simulink model "EHB_MOTOR"  (R2023b)
settings: Solver=FixedStepDiscrete  StartTime=0.0  StopTime=inf  FixedStep=0.0001  RelTol=1e-3  EnableMultiTasking=on
undefined symbols (not defined in the file): CAN_EHB_VCU0x125, CAN_EHB_VCU0x126, CAN_id0x120_Data, Cos_Table, Cos_Table1, EHB_DTC_status, R, Sin_BreakPoint, Sin_BreakPoint1, Sin_Table, Sin_Table1, T
libraries: simulink x30
(part 8 of 9)

== stateflow chart EHB_MOTOR/EHB_MOTOR_PRO/DIAG/MotLockDiag/ErrorSignalCount ==
  state errClear
    en:Mot_locked_err=0;
    Counter=0;
  state errConfirm
    en:Mot_locked_err=0;
    du:Counter++;
  state errTrue
    en:Mot_locked_err=1;
    Counter=0;
  (default) -> errClear
  errClear -> errConfirm : [Mot_locked==1]
  errConfirm -> errClear [order 2] : [Mot_locked==0]
  errTrue -> errClear : [Recover==1]
  errConfirm -> errTrue [order 1] : [Counter >= tiMotLocked_C]
  data: Mot_locked input boolean; Mot_locked_err output boolean; tiMotLocked_C input uint16; Counter local uint16; Recover input uint8

== stateflow chart EHB_MOTOR/EHB_MOTOR_PRO/MODE/Chart1 ==
  (default) -> (junction 5)
  (junction 5) -> (junction 7) [order 1] : [input]
  (junction 5) -> (junction 23) [order 2] : {ZeroCal_cnt=0;}
  (junction 7) -> (junction 9) : {ZeroCal_cnt++;}
  (junction 9) -> (junction 13) [order 1] : [ZeroCal_cnt>=9000]
  (junction 9) -> (junction 20) [order 2]
  (junction 13) -> (junction 15) : {Zero_Angle=MOT_Angle;
      | ZeroCal_cmplt=1;}
  (junction 20) -> (junction 23)
  (junction 15) -> (junction 20)
  data: MOT_Angle input uint16; input input boolean; ZeroCal_cnt local uint16; Zero_Angle output uint16; ZeroCal_cmplt output boolean

== stateflow chart EHB_MOTOR/EHB_MOTOR_PRO/DIAG/UDS_interface/DTC_pack ==
  (default) -> (junction 15) : %12v欠压故障
  (junction 15) -> (junction 17) [order 1] : [minBAT == 1]
  (junction 15) -> (junction 25) [order 2] : {EHB_DTC[12]&=0x01;}
  (junction 17) -> (junction 20) : {EHB_DTC[12]|=0x03;}
  (junction 25) -> (junction 20)
  (junction 20) -> (junction 30) [order 1] : [Clear_minBAT_req == 1]
  (junction 20) -> (junction 34) [order 2]
  (junction 30) -> (junction 32) : {EHB_DTC[12]&=0x02;}
  (junction 34) -> (junction 32)
  (junction 32) -> (junction 66) : %12v过压故障
  (junction 66) -> (junction 68) [order 1] : [maxBAT == 1]
  (junction 66) -> (junction 72) [order 2] : {EHB_DTC[13]&=0x01;}
  (junction 68) -> (junction 70) : {EHB_DTC[13]|=0x03;}
  (junction 72) -> (junction 70)
  (junction 70) -> (junction 78) [order 1] : [Clear_minBAT_req == 1]
  (junction 70) -> (junction 80) [order 2]
  (junction 78) -> (junction 75) : {EHB_DTC[13]&=0x02;}
  (junction 80) -> (junction 75)
  (junction 75) -> (junction 97) : %过温故障
  (junction 97) -> (junction 91) [order 1] : [overTemp == 1]
  (junction 97) -> (junction 95) [order 2] : {EHB_DTC[10]&=0x01;}
  (junction 91) -> (junction 89) : {EHB_DTC[10]|=0x03;}
  (junction 95) -> (junction 89)
  (junction 89) -> (junction 87) [order 1] : [Clear_minBAT_req == 1]
  (junction 89) -> (junction 83) [order 2]
  (junction 87) -> (junction 94) : {EHB_DTC[10]&=0x02;}
  (junction 83) -> (junction 94)
  (junction 94) -> (junction 103) : %温度传感器故障
  (junction 103) -> (junction 108) [order 1] : [errTempSensor == 1]
  (junction 103) -> (junction 106) [order 2] : {EHB_DTC[15]&=0x01;}
  (junction 108) -> (junction 105) : {EHB_DTC[15]|=0x03;}
  (junction 106) -> (junction 105)
  (junction 105) -> (junction 112) [order 1] : [Clear_minBAT_req == 1]
  (junction 105) -> (junction 115) [order 2]
  (junction 112) -> (junction 104) : {EHB_DTC[15]&=0x02;}
  (junction 115) -> (junction 104)
  (junction 104) -> (junction 127) : %过流故障
  (junction 127) -> (junction 131) [order 1] : [overCurrent == 1]
  (junction 127) -> (junction 124) [order 2] : {EHB_DTC[11]&=0x01;}
  (junction 131) -> (junction 118) : {EHB_DTC[11]|=0x03;}
  (junction 124) -> (junction 118)
  (junction 118) -> (junction 123) [order 1] : [Clear_minBAT_req == 1]
  (junction 118) -> (junction 129) [order 2]
  (junction 123) -> (junction 128) : {EHB_DTC[11]&=0x02;}
  (junction 129) -> (junction 128)
  (junction 128) -> (junction 140) : %电流传感器故障
  (junction 140) -> (junction 145) [order 1] : [errCurSensor == 1]
  (junction 140) -> (junction 148) [order 2] : {EHB_DTC[14]&=0x01;}
  (junction 145) -> (junction 138) : {EHB_DTC[14]|=0x03;}
  (junction 148) -> (junction 138)
  (junction 138) -> (junction 135) [order 1] : [Clear_minBAT_req == 1]
  (junction 138) -> (junction 141) [order 2]
  (junction 135) -> (junction 147) : {EHB_DTC[14]&=0x02;}
  (junction 141) -> (junction 147)
  (junction 147) -> (junction 162) : %角度传感器信号错误故障
  (junction 162) -> (junction 151) [order 1] : [errAngleSensor == 1]
  (junction 162) -> (junction 153) [order 2] : {EHB_DTC[0]&=0x01;}
  (junction 151) -> (junction 157) : {EHB_DTC[0]|=0x03;}
  (junction 153) -> (junction 157)
  (junction 157) -> (junction 164) [order 1] : [Clear_minBAT_req == 1]
  (junction 157) -> (junction 154) [order 2]
  (junction 164) -> (junction 150) : {EHB_DTC[0]&=0x02;}
  (junction 154) -> (junction 150)
  (junction 150) -> (junction 168) : %角度传感器没有信号故障
  (junction 168) -> (junction 175) [order 1] : [noAngleSensor == 1]
  (junction 168) -> (junction 173) [order 2] : {EHB_DTC[1]&=0x01;}
  (junction 175) -> (junction 169) : {EHB_DTC[1]|=0x03;}
  (junction 173) -> (junction 169)
  (junction 169) -> (junction 174) [order 1] : [Clear_minBAT_req == 1]
  (junction 169) -> (junction 176) [order 2]
  (junction 174) -> (junction 180) : {EHB_DTC[1]&=0x02;}
  (junction 176) -> (junction 180)
  (junction 180) -> (junction 183) : %角度传感器没有标定故障
  (junction 183) -> (junction 193) [order 1] : [unCalAngleSensor == 1]
  (junction 183) -> (junction 195) [order 2] : {EHB_DTC[2]&=0x01;}
  (junction 193) -> (junction 185) : {EHB_DTC[2]|=0x03;}
  (junction 195) -> (junction 185)
  (junction 185) -> (junction 188) [order 1] : [Clear_minBAT_req == 1]
  (junction 185) -> (junction 190) [order 2]
  (junction 188) -> (junction 191) : {EHB_DTC[2]&=0x02;}
  (junction 190) -> (junction 191)
  (junction 191) -> (junction 208) : %压力传感器信号错误故障
  (junction 208) -> (junction 205) [order 1] : [errPreSensor == 1]
  (junction 208) -> (junction 198) [order 2] : {EHB_DTC[3]&=0x01;}
  (junction 205) -> (junction 209) : {EHB_DTC[3]|=0x03;}
  (junction 198) -> (junction 209)
  (junction 209) -> (junction 200) [order 1] : [Clear_minBAT_req == 1]
  (junction 209) -> (junction 207) [order 2]
  (junction 200) -> (junction 199) : {EHB_DTC[3]&=0x02;}
  (junction 207) -> (junction 199)
  (junction 199) -> (junction 218) : %压力传感器没有信号故障
  (junction 218) -> (junction 216) [order 1] : [noPreSensor == 1]
  (junction 218) -> (junction 228) [order 2] : {EHB_DTC[4]&=0x01;}
  (junction 216) -> (junction 215) : {EHB_DTC[4]|=0x03;}
  (junction 228) -> (junction 215)
  (junction 215) -> (junction 224) [order 1] : [Clear_minBAT_req == 1]
  (junction 215) -> (junction 221) [order 2]
  (junction 224) -> (junction 220) : {EHB_DTC[4]&=0x02;}
  (junction 221) -> (junction 220)
  (junction 220) -> (junction 238) : %压力传感器没有标定故障
  (junction 238) -> (junction 235) [order 1] : [unCalPreSensor == 1]
  (junction 238) -> (junction 230) [order 2] : {EHB_DTC[5]&=0x01;}
  (junction 235) -> (junction 239) : {EHB_DTC[5]|=0x03;}
  (junction 230) -> (junction 239)
  (junction 239) -> (junction 233) [order 1] : [Clear_minBAT_req == 1]
  (junction 239) -> (junction 234) [order 2]
  (junction 233) -> (junction 242) : {EHB_DTC[5]&=0x02;}
  (junction 234) -> (junction 242)
  (junction 242) -> (junction 248) : %扭矩传感器信号错误故障
  (junction 248) -> (junction 256) [order 1] : [errTqSensor == 1]
  (junction 248) -> (junction 259) [order 2] : {EHB_DTC[6]&=0x01;}
  (junction 256) -> (junction 251) : {EHB_DTC[6]|=0x03;}
  (junction 259) -> (junction 251)
  (junction 251) -> (junction 257) [order 1] : [Clear_minBAT_req == 1]
  (junction 251) -> (junction 252) [order 2]
  (junction 257) -> (junction 246) : {EHB_DTC[6]&=0x02;}
  (junction 252) -> (junction 246)
  (junction 246) -> (junction 276) : %扭矩传感器没有信号故障
  (junction 276) -> (junction 273) [order 1] : [noTqSensor == 1]
  (junction 276) -> (junction 268) [order 2] : {EHB_DTC[7]&=0x01;}
  (junction 273) -> (junction 269) : {EHB_DTC[7]|=0x03;}
  (junction 268) -> (junction 269)
  (junction 269) -> (junction 264) [order 1] : [Clear_minBAT_req == 1]
  (junction 269) -> (junction 270) [order 2]
  (junction 264) -> (junction 274) : {EHB_DTC[7]&=0x02;}
  (junction 270) -> (junction 274)
  (junction 274) -> (junction 289) : %扭矩传感器没有标定故障
  (junction 289) -> (junction 279) [order 1] : [unCalTqSensor == 1]
  (junction 289) -> (junction 288) [order 2] : {EHB_DTC[8]&=0x01;}
  (junction 279) -> (junction 285) : {EHB_DTC[8]|=0x03;}
  (junction 288) -> (junction 285)
  (junction 285) -> (junction 290) [order 1] : [Clear_minBAT_req == 1]
  (junction 285) -> (junction 283) [order 2]
  (junction 290) -> (junction 280) : {EHB_DTC[8]&=0x02;}
  (junction 283) -> (junction 280)
  (junction 280) -> (junction 295) : %电机回路故障
  (junction 295) -> (junction 304) [order 1] : [errMotorloop == 1]
  (junction 295) -> (junction 305) [order 2] : {EHB_DTC[9]&=0x01;}
  (junction 304) -> (junction 298) : {EHB_DTC[9]|=0x03;}
  (junction 305) -> (junction 298)
  (junction 298) -> (junction 297) [order 1] : [Clear_minBAT_req == 1]
  (junction 298) -> (junction 299) [order 2]
  (junction 297) -> (junction 306) : {EHB_DTC[9]&=0x02;}
  (junction 299) -> (junction 306)
  (junction 306) -> (junction 323) : %预充电路故障
  (junction 323) -> (junction 316) [order 1] : [errPreCtl == 1]
  (junction 323) -> (junction 315) [order 2] : {EHB_DTC[16]&=0x01;}
  (junction 316) -> (junction 318) : {EHB_DTC[16]|=0x03;}
  (junction 315) -> (junction 318)
  (junction 318) -> (junction 321) [order 1] : [Clear_minBAT_req == 1]
  (junction 318) -> (junction 314) [order 2]
  (junction 321) -> (junction 319) : {EHB_DTC[16]&=0x02;}
  (junction 314) -> (junction 319)
  (junction 319) -> (junction 326) : %5v输出电路故障
  (junction 326) -> (junction 337) [order 1] : [err5vOUT == 1]
  (junction 326) -> (junction 335) [order 2] : {EHB_DTC[17]&=0x01;}
  (junction 337) -> (junction 333) : {EHB_DTC[17]|=0x03;}
  (junction 335) -> (junction 333)
  (junction 333) -> (junction 329) [order 1] : [Clear_minBAT_req == 1]
  (junction 333) -> (junction 334) [order 2]
  (junction 329) -> (junction 328) : {EHB_DTC[17]&=0x02;}
  (junction 334) -> (junction 328)
  (junction 328) -> (junction 356) : %高边输出电路1故障
  (junction 356) -> (junction 348) [order 1] : [errHSO1 == 1]
  (junction 356) -> (junction 352) [order 2] : {EHB_DTC[18]&=0x01;}
  (junction 348) -> (junction 349) : {EHB_DTC[18]|=0x03;}
  (junction 352) -> (junction 349)
  (junction 349) -> (junction 346) [order 1] : [Clear_minBAT_req == 1]
  (junction 349) -> (junction 345) [order 2]
  (junction 346) -> (junction 350) : {EHB_DTC[18]&=0x02;}
  (junction 345) -> (junction 350)
  (junction 350) -> (junction 358) : %高边输出电路2故障
  (junction 358) -> (junction 363) [order 1] : [errHSO2 == 1]
  (junction 358) -> (junction 368) [order 2] : {EHB_DTC[19]&=0x01;}
  (junction 363) -> (junction 371) : {EHB_DTC[19]|=0x03;}
  (junction 368) -> (junction 371)
  (junction 371) -> (junction 372) [order 1] : [Clear_minBAT_req == 1]
  (junction 371) -> (junction 366) [order 2]
  (junction 372) -> (junction 362) : {EHB_DTC[19]&=0x02;}
  (junction 366) -> (junction 362)
  (junction 362) -> (junction 386) : %A3941芯片故障
  (junction 386) -> (junction 382) [order 1] : [errA3941 == 1]
  (junction 386) -> (junction 376) [order 2] : {EHB_DTC[20]&=0x01;}
  (junction 382) -> (junction 377) : {EHB_DTC[20]|=0x03;}
  (junction 376) -> (junction 377)
  (junction 377) -> (junction 388) [order 1] : [Clear_minBAT_req == 1]
  (junction 377) -> (junction 379) [order 2]
  (junction 388) -> (junction 385) : {EHB_DTC[20]&=0x02;}
  (junction 379) -> (junction 385)
  (junction 385) -> (junction 392) : %占空比发送电路故障
  (junction 392) -> (junction 403) [order 1] : [errPWM == 1]
  (junction 392) -> (junction 404) [order 2] : {EHB_DTC[21]&=0x01;}
  (junction 403) -> (junction 394) : {EHB_DTC[21]|=0x03;}
  (junction 404) -> (junction 394)
  (junction 394) -> (junction 390) [order 1] : [Clear_minBAT_req == 1]
  (junction 394) -> (junction 393) [order 2]
  (junction 390) -> (junction 397) : {EHB_DTC[21]&=0x02;}
  (junction 393) -> (junction 397)
  (junction 397) -> (junction 419) : %电机响应状态异常故障
  (junction 419) -> (junction 406) [order 1] : [errResponce == 1]
  (junction 419) -> (junction 418) [order 2] : {EHB_DTC[22]&=0x01;}
  (junction 406) -> (junction 409) : {EHB_DTC[22]|=0x03;}
  (junction 418) -> (junction 409)
  (junction 409) -> (junction 420) [order 1] : [Clear_minBAT_req == 1]
  (junction 409) -> (junction 408) [order 2]
  (junction 420) -> (junction 410) : {EHB_DTC[22]&=0x02;}
  (junction 408) -> (junction 410)
  (junction 410) -> (junction 422) : %CAN收发器电路故障
  (junction 422) -> (junction 434) [order 1] : [errCANHW == 1]
  (junction 422) -> (junction 423) [order 2] : {EHB_DTC[23]&=0x01;}
  (junction 434) -> (junction 430) : {EHB_DTC[23]|=0x03;}
  (junction 423) -> (junction 430)
  (junction 430) -> (junction 436) [order 1] : [Clear_minBAT_req == 1]
  (junction 430) -> (junction 429) [order 2]
  (junction 436) -> (junction 425) : {EHB_DTC[23]&=0x02;}
  (junction 429) -> (junction 425)
  (junction 425) -> (junction 442) : %CAN数据丢失故障
  (junction 442) -> (junction 446) [order 1] : [CANDataLoss == 1]
  (junction 442) -> (junction 440) [order 2] : {EHB_DTC[24]&=0x01;}
  (junction 446) -> (junction 451) : {EHB_DTC[24]|=0x03;}
  (junction 440) -> (junction 451)
  (junction 451) -> (junction 450) [order 1] : [Clear_minBAT_req == 1]
  (junction 451) -> (junction 445) [order 2]
  (junction 450) -> (junction 438) : {EHB_DTC[24]&=0x02;}
  (junction 445) -> (junction 438)
  (junction 438) -> (junction 462) : %CAN BUSOFF
  (junction 462) -> (junction 466) [order 1] : [BUSOFF == 1]
  (junction 462) -> (junction 468) [order 2] : {EHB_DTC[25]&=0x01;}
  (junction 466) -> (junction 455) : {EHB_DTC[25]|=0x03;}
  (junction 468) -> (junction 455)
  (junction 455) -> (junction 456) [order 1] : [Clear_minBAT_req == 1]
  (junction 455) -> (junction 459) [order 2]
  (junction 456) -> (junction 463) : {EHB_DTC[25]&=0x02;}
  (junction 459) -> (junction 463)
  (junction 463) -> (junction 476) : %Tracker2对地短路故障
  (junction 476) -> (junction 506) [order 1] : [Tracker2_Short2GND_err == 1]
  (junction 476) -> (junction 520) [order 2] : {EHB_DTC[26]&=0x01;}
  (junction 506) -> (junction 474) : {EHB_DTC[26]|=0x03;}
  (junction 520) -> (junction 474)
  (junction 474) -> (junction 511) [order 1] : [Clear_minBAT_req == 1]
  (junction 474) -> (junction 499) [order 2]
  (junction 511) -> (junction 473) : {EHB_DTC[26]&=0x02;}
  (junction 499) -> (junction 473)
  (junction 473) -> (junction 522) : %Tracker2过压故障
  (junction 522) -> (junction 518) [order 1] : [Tracker2_OverVolt_err == 1]
  (junction 522) -> (junction 519) [order 2] : {EHB_DTC[27]&=0x01;}
  (junction 518) -> (junction 500) : {EHB_DTC[27]|=0x03;}
  (junction 519) -> (junction 500)
  (junction 500) -> (junction 501) [order 1] : [Clear_minBAT_req == 1]
  (junction 500) -> (junction 510) [order 2]
  (junction 501) -> (junction 471) : {EHB_DTC[27]&=0x02;}
  (junction 510) -> (junction 471)
  (junction 471) -> (junction 515) : %Tracker2欠压故障
  (junction 515) -> (junction 512) [order 1] : [Tracker2_UnderVolt_err == 1]
  (junction 515) -> (junction 502) [order 2] : {EHB_DTC[28]&=0x01;}
  (junction 512) -> (junction 503) : {EHB_DTC[28]|=0x03;}
  (junction 502) -> (junction 503)
  (junction 503) -> (junction 472) [order 1] : [Clear_minBAT_req == 1]
  (junction 503) -> (junction 514) [order 2]
  (junction 472) -> (junction 484) : {EHB_DTC[28]&=0x02;}
  (junction 514) -> (junction 484)
  (junction 484) -> (junction 509) : %Tracker1对地短路故障
  (junction 509) -> (junction 513) [order 1] : [Tracker1_Short2GND_err == 1]
  (junction 509) -> (junction 521) [order 2] : {EHB_DTC[29]&=0x01;}
  (junction 513) -> (junction 508) : {EHB_DTC[29]|=0x03;}
  (junction 521) -> (junction 508)
  (junction 508) -> (junction 523) [order 1] : [Clear_minBAT_req == 1]
  (junction 508) -> (junction 491) [order 2]
  (junction 523) -> (junction 516) : {EHB_DTC[29]&=0x02;}
  (junction 491) -> (junction 516)
  (junction 516) -> (junction 517) : %Tracker1过压故障
  (junction 517) -> (junction 504) [order 1] : [Tracker1_OverVolt_err == 1]
  (junction 517) -> (junction 524) [order 2] : {EHB_DTC[30]&=0x01;}
  (junction 504) -> (junction 470) : {EHB_DTC[30]|=0x03;}
  (junction 524) -> (junction 470)
  (junction 470) -> (junction 494) [order 1] : [Clear_minBAT_req == 1]
  (junction 470) -> (junction 505) [order 2]
  (junction 494) -> (junction 496) : {EHB_DTC[30]&=0x02;}
  (junction 505) -> (junction 496)
  (junction 496) -> (junction 485) : %Tracker1欠压故障
  (junction 485) -> (junction 507) [order 1] : [Tracker1_UnderVolt_err == 1]
  (junction 485) -> (junction 475) [order 2] : {EHB_DTC[31]&=0x01;}
  (junction 507) -> (junction 492) : {EHB_DTC[31]|=0x03;}
  (junction 475) -> (junction 492)
  (junction 492) -> (junction 477) [order 1] : [Clear_minBAT_req == 1]
  (junction 492) -> (junction 478) [order 2]
  (junction 477) -> (junction 479) : {EHB_DTC[31]&=0x02;}
  (junction 478) -> (junction 479)
  (junction 479) -> (junction 480) : %Voltage reference对地短路故障
  (junction 480) -> (junction 481) [order 1] : [VltRef_Short2GND_err == 1]
  (junction 480) -> (junction 497) [order 2] : {EHB_DTC[32]&=0x01;}
  (junction 481) -> (junction 482) : {EHB_DTC[32]|=0x03;}
  (junction 497) -> (junction 482)
  (junction 482) -> (junction 486) [order 1] : [Clear_minBAT_req == 1]
  (junction 482) -> (junction 483) [order 2]
  (junction 486) -> (junction 487) : {EHB_DTC[32]&=0x02;}
  (junction 483) -> (junction 487)
  (junction 487) -> (junction 493) : %Voltage reference过压故障
  (junction 493) -> (junction 488) [order 1] : [VltRef_OverVolt_err == 1]
  (junction 493) -> (junction 489) [order 2] : {EHB_DTC[33]&=0x01;}
  (junction 488) -> (junction 490) : {EHB_DTC[33]|=0x03;}
  (junction 489) -> (junction 490)
  (junction 490) -> (junction 495) [order 1] : [Clear_minBAT_req == 1]
  (junction 490) -> (junction 498) [order 2]
  (junction 495) -> (junction 553) : {EHB_DTC[33]&=0x02;}
  (junction 498) -> (junction 553)
  (junction 553) -> (junction 537) : %Voltage reference欠压故障
  (junction 537) -> (junction 554) [order 1] : [VltRef_UnderVolt_err == 1]
  (junction 537) -> (junction 587) [order 2] : {EHB_DTC[34]&=0x01;}
  (junction 554) -> (junction 582) : {EHB_DTC[34]|=0x03;}
  (junction 587) -> (junction 582)
  (junction 582) -> (junction 576) [order 1] : [Clear_minBAT_req == 1]
  (junction 582) -> (junction 539) [order 2]
  (junction 576) -> (junction 568) : {EHB_DTC[34]&=0x02;}
  (junction 539) -> (junction 568)
  (junction 568) -> (junction 556) : %Communication LDO对地短路故障
  (junction 556) -> (junction 583) [order 1] : [CommuLDO_Short2GND_err == 1]
  (junction 556) -> (junction 541) [order 2] : {EHB_DTC[35]&=0x01;}
  (junction 583) -> (junction 562) : {EHB_DTC[35]|=0x03;}
  (junction 541) -> (junction 562)
  (junction 562) -> (junction 555) [order 1] : [Clear_minBAT_req == 1]
  (junction 562) -> (junction 560) [order 2]
  (junction 555) -> (junction 532) : {EHB_DTC[35]&=0x02;}
  (junction 560) -> (junction 532)
  (junction 532) -> (junction 579) : %Communication LDO过压故障
  (junction 579) -> (junction 540) [order 1] : [CommuLDO_OverVolt_err == 1]
  (junction 579) -> (junction 558) [order 2] : {EHB_DTC[36]&=0x01;}
  (junction 540) -> (junction 570) : {EHB_DTC[36]|=0x03;}
  (junction 558) -> (junction 570)
  (junction 570) -> (junction 584) [order 1] : [Clear_minBAT_req == 1]
  (junction 570) -> (junction 561) [order 2]
  (junction 584) -> (junction 557) : {EHB_DTC[36]&=0x02;}
  (junction 561) -> (junction 557)
  (junction 557) -> (junction 552) : %Communication LDO欠压故障
  (junction 552) -> (junction 547) [order 1] : [CommuLDO_UnderVolt_err == 1]
  (junction 552) -> (junction 563) [order 2] : {EHB_DTC[37]&=0x01;}
  (junction 547) -> (junction 559) : {EHB_DTC[37]|=0x03;}
  (junction 563) -> (junction 559)
  (junction 559) -> (junction 564) [order 1] : [Clear_minBAT_req == 1]
  (junction 559) -> (junction 573) [order 2]
  (junction 564) -> (junction 586) : {EHB_DTC[37]&=0x02;}
  (junction 573) -> (junction 586)
  (junction 586) -> (junction 535) : %Core voltage对地短路故障
  (junction 535) -> (junction 581) [order 1] : [CoreVlt_Short2GND_err == 1]
  (junction 535) -> (junction 585) [order 2] : {EHB_DTC[38]&=0x01;}
  (junction 581) -> (junction 549) : {EHB_DTC[38]|=0x03;}
  (junction 585) -> (junction 549)
  (junction 549) -> (junction 565) [order 1] : [Clear_minBAT_req == 1]
  (junction 549) -> (junction 551) [order 2]
  (junction 565) -> (junction 542) : {EHB_DTC[38]&=0x02;}
  (junction 551) -> (junction 542)
  (junction 542) -> (junction 566) : %Core voltage过压故障
  (junction 566) -> (junction 528) [order 1] : [CoreVlt_OverVolt_err == 1]
  (junction 566) -> (junction 546) [order 2] : {EHB_DTC[39]&=0x01;}
  (junction 528) -> (junction 567) : {EHB_DTC[39]|=0x03;}
  (junction 546) -> (junction 567)
  (junction 567) -> (junction 574) [order 1] : [Clear_minBAT_req == 1]
  (junction 567) -> (junction 569) [order 2]
  (junction 574) -> (junction 588) : {EHB_DTC[39]&=0x02;}
  (junction 569) -> (junction 588)
  (junction 588) -> (junction 571) : %Core voltage欠压故障
  (junction 571) -> (junction 572) [order 1] : [CoreVlt_UnderVolt_err == 1]
  (junction 571) -> (junction 575) [order 2] : {EHB_DTC[40]&=0x01;}
  (junction 572) -> (junction 577) : {EHB_DTC[40]|=0x03;}
  (junction 575) -> (junction 577)
  (junction 577) -> (junction 578) [order 1] : [Clear_minBAT_req == 1]
  (junction 577) -> (junction 533) [order 2]
  (junction 578) -> (junction 580) : {EHB_DTC[40]&=0x02;}
  (junction 533) -> (junction 580)
  (junction 580) -> (junction 525) : %Standby LDO对地短路故障
  (junction 525) -> (junction 526) [order 1] : [StdbyLDO_Short2GND_err == 1]
  (junction 525) -> (junction 527) [order 2] : {EHB_DTC[41]&=0x01;}
  (junction 526) -> (junction 529) : {EHB_DTC[41]|=0x03;}
  (junction 527) -> (junction 529)
  (junction 529) -> (junction 530) [order 1] : [Clear_minBAT_req == 1]
  (junction 529) -> (junction 531) [order 2]
  (junction 530) -> (junction 534) : {EHB_DTC[41]&=0x02;}
  (junction 531) -> (junction 534)
  (junction 534) -> (junction 536) : %Standby LDO过压故障
  (junction 536) -> (junction 538) [order 1] : [StdbyLDO_OverVolt_err == 1]
  (junction 536) -> (junction 543) [order 2] : {EHB_DTC[42]&=0x01;}
  (junction 538) -> (junction 544) : {EHB_DTC[42]|=0x03;}
  (junction 543) -> (junction 544)
  (junction 544) -> (junction 545) [order 1] : [Clear_minBAT_req == 1]
  (junction 544) -> (junction 548) [order 2]
  (junction 545) -> (junction 550) : {EHB_DTC[42]&=0x02;}
  (junction 548) -> (junction 550)
  (junction 550) -> (junction 615) : %Standby LDO欠压故障
  (junction 615) -> (junction 614) [order 1] : [StdbyLDO_UnderVolt_err == 1]
  (junction 615) -> (junction 608) [order 2] : {EHB_DTC[43]&=0x01;}
  (junction 614) -> (junction 599) : {EHB_DTC[43]|=0x03;}
  (junction 608) -> (junction 599)
  (junction 599) -> (junction 602) [order 1] : [Clear_minBAT_req == 1]
  (junction 599) -> (junction 616) [order 2]
  (junction 602) -> (junction 623) : {EHB_DTC[43]&=0x02;}
  (junction 616) -> (junction 623)
  (junction 623) -> (junction 620) : %uC LDO对地短路故障
  (junction 620) -> (junction 632) [order 1] : [uCLDO_Short2GND_err == 1]
  (junction 620) -> (junction 617) [order 2] : {EHB_DTC[44]&=0x01;}
  (junction 632) -> (junction 633) : {EHB_DTC[44]|=0x03;}
  (junction 617) -> (junction 633)
  (junction 633) -> (junction 619) [order 1] : [Clear_minBAT_req == 1]
  (junction 633) -> (junction 605) [order 2]
  (junction 619) -> (junction 594) : {EHB_DTC[44]&=0x02;}
  (junction 605) -> (junction 594)
  (junction 594) -> (junction 589) : %uC LDO过压故障
  (junction 589) -> (junction 624) [order 1] : [uCLDO_OverVolt_err == 1]
  (junction 589) -> (junction 593) [order 2] : {EHB_DTC[45]&=0x01;}
  (junction 624) -> (junction 612) : {EHB_DTC[45]|=0x03;}
  (junction 593) -> (junction 612)
  (junction 612) -> (junction 596) [order 1] : [Clear_minBAT_req == 1]
  (junction 612) -> (junction 600) [order 2]
  (junction 596) -> (junction 595) : {EHB_DTC[45]&=0x02;}
  (junction 600) -> (junction 595)
  (junction 595) -> (junction 592) : %uC LDO欠压故障
  (junction 592) -> (junction 622) [order 1] : [uCLDO_UnderVolt_err == 1]
  (junction 592) -> (junction 610) [order 2] : {EHB_DTC[46]&=0x01;}
  (junction 622) -> (junction 618) : {EHB_DTC[46]|=0x03;}
  (junction 610) -> (junction 618)
  (junction 618) -> (junction 636) [order 1] : [Clear_minBAT_req == 1]
  (junction 618) -> (junction 625) [order 2]
  (junction 636) -> (junction 590) : {EHB_DTC[46]&=0x02;}
  (junction 625) -> (junction 590)
  (junction 590) -> (junction 627) : %Pre-regulator voltage对地短路故障
  (junction 627) -> (junction 621) [order 1] : [PreVolt_Short2GND_err == 1]
  (junction 627) -> (junction 609) [order 2] : {EHB_DTC[47]&=0x01;}
  (junction 621) -> (junction 611) : {EHB_DTC[47]|=0x03;}
  (junction 609) -> (junction 611)
  (junction 611) -> (junction 603) [order 1] : [Clear_minBAT_req == 1]
  (junction 611) -> (junction 601) [order 2]
  (junction 603) -> (junction 626) : {EHB_DTC[47]&=0x02;}
  (junction 601) -> (junction 626)
  (junction 626) -> (junction 606) : %Pre-regulator voltage过压故障
  (junction 606) -> (junction 597) [order 1] : [PreVolt_OverVolt_err == 1]
  (junction 606) -> (junction 607) [order 2] : {EHB_DTC[48]&=0x01;}
  (junction 597) -> (junction 637) : {EHB_DTC[48]|=0x03;}
  (junction 607) -> (junction 637)
  (junction 637) -> (junction 634) [order 1] : [Clear_minBAT_req == 1]
  (junction 637) -> (junction 628) [order 2]
  (junction 634) -> (junction 598) : {EHB_DTC[48]&=0x02;}
  (junction 628) -> (junction 598)
  (junction 598) -> (junction 629) : %Pre-regulator voltage欠压故障
  (junction 629) -> (junction 630) [order 1] : [PreVolt_UnderVolt_err == 1]
  (junction 629) -> (junction 631) [order 2] : {EHB_DTC[49]&=0x01;}
  (junction 630) -> (junction 635) : {EHB_DTC[49]|=0x03;}
  (junction 631) -> (junction 635)
  (junction 635) -> (junction 591) [order 1] : [Clear_minBAT_req == 1]
  (junction 635) -> (junction 638) [order 2]
  (junction 591) -> (junction 604) : {EHB_DTC[49]&=0x02;}
  (junction 638) -> (junction 604)
  data: minBAT input; maxBAT input; EHB_DTC output uint8 size=50; overTemp input; errTempSensor input; overCurrent input; errCurSensor input; errAngleSensor input; noAngleSensor input; unCalAngleSensor input; errPreSensor input; noPreSensor input; unCalPreSensor input; errTqSensor input; noTqSensor input; unCalTqSensor input; errMotorloop input; errPreCtl input; err5vOUT input; errHSO1 input; errHSO2 input; errA3941 input; errPWM input; errResponce input; errCANHW input; CANDataLoss input; BUSOFF input; Clear_minBAT_req input; Tracker2_Short2GND_err input; Tracker2_OverVolt_err input; Tracker2_UnderVolt_err input; Tracker1_Short2GND_err input; Tracker1_OverVolt_err input; Tracker1_UnderVolt_err input; VltRef_Short2GND_err input; VltRef_OverVolt_err input; VltRef_UnderVolt_err input; CommuLDO_Short2GND_err input; CommuLDO_OverVolt_err input; CommuLDO_UnderVolt_err input; CoreVlt_Short2GND_err input; CoreVlt_OverVolt_err input; CoreVlt_UnderVolt_err input; StdbyLDO_Short2GND_err input; StdbyLDO_OverVolt_err input; StdbyLDO_UnderVolt_err input; uCLDO_Short2GND_err input; uCLDO_OverVolt_err input; uCLDO_UnderVolt_err input; PreVolt_Short2GND_err input; PreVolt_OverVolt_err input; PreVolt_UnderVolt_err input

== stateflow chart EHB_MOTOR/EHB_MOTOR_PRO/DIAG/TLF35584Diag/ErrorSignalCount ==
  state errConfirm
    en:Tracker2_Short2GND_err=0;
    du:Counter++;
  state errClear
    en:Tracker2_Short2GND_err=0;
    Counter=0;
  state errTrue
    en:Tracker2_Short2GND_err=1;
    Counter=0;
  (default) -> errClear
  errClear -> errConfirm : [TLF35584Tracker2_Short2GND==1]
  errConfirm -> errClear [order 2] : [TLF35584Tracker2_Short2GND==0]
  errTrue -> errClear : [Recover==1]
  errConfirm -> errTrue [order 1] : [Counter >= ti35584err_C]
  data: TLF35584Tracker2_Short2GND input boolean; Tracker2_Short2GND_err output boolean; ti35584err_C input uint16; Counter local uint16; Recover input uint8

== stateflow chart EHB_MOTOR/EHB_MOTOR_PRO/DIAG/TLF35584Diag/ErrorSignalCount1 ==
  state errConfirm
    en:Tracker1_Short2GND_err=0;
    du:Counter++;
  state errClear
    en:Tracker1_Short2GND_err=0;
    Counter=0;
  state errTrue
    en:Tracker1_Short2GND_err=1;
    Counter=0;
  (default) -> errClear
  errClear -> errConfirm : [TLF35584Tracker1_Short2GND==1]
  errConfirm -> errClear [order 2] : [TLF35584Tracker1_Short2GND==0]
  errTrue -> errClear : [Recover==1]
  errConfirm -> errTrue [order 1] : [Counter >= ti35584err_C]
  data: TLF35584Tracker1_Short2GND input boolean; Tracker1_Short2GND_err output boolean; ti35584err_C input uint16; Counter local uint16; Recover input uint8

== stateflow chart EHB_MOTOR/EHB_MOTOR_PRO/DIAG/TLF35584Diag/ErrorSignalCount2 ==
  state errConfirm
    en:Tracker2_OverVolt_err=0;
    du:Counter++;
  state errClear
    en:Tracker2_OverVolt_err=0;
    Counter=0;
  state errTrue
    en:Tracker2_OverVolt_err=1;
    Counter=0;
  (default) -> errClear
  errClear -> errConfirm : [TLF35584Tracker2_OverVolt==1]
  errConfirm -> errClear [order 2] : [TLF35584Tracker2_OverVolt==0]
  errTrue -> errClear : [Recover==1]
  errConfirm -> errTrue [order 1] : [Counter >= ti35584err_C]
  data: TLF35584Tracker2_OverVolt input boolean; Tracker2_OverVolt_err output boolean; ti35584err_C input uint16; Counter local uint16; Recover input uint8

== stateflow chart EHB_MOTOR/EHB_MOTOR_PRO/DIAG/TLF35584Diag/ErrorSignalCount3 ==
  state errConfirm
    en:Tracker2_UnderVolt_err=0;
    du:Counter++;
  state errClear
    en:Tracker2_UnderVolt_err=0;
    Counter=0;
  state errTrue
    en:Tracker2_UnderVolt_err=1;
    Counter=0;
  (default) -> errClear
  errClear -> errConfirm : [TLF35584Tracker2_UnderVolt==1]
  errConfirm -> errClear [order 2] : [TLF35584Tracker2_UnderVolt==0]
  errTrue -> errClear : [Recover==1]
  errConfirm -> errTrue [order 1] : [Counter >= ti35584err_C]
  data: TLF35584Tracker2_UnderVolt input boolean; Tracker2_UnderVolt_err output boolean; ti35584err_C input uint16; Counter local uint16; Recover input uint8

== stateflow chart EHB_MOTOR/EHB_MOTOR_PRO/DIAG/TLF35584Diag/ErrorSignalCount4 ==
  state errConfirm
    en:Tracker1_OverVolt_err=0;
    du:Counter++;
  state errClear
    en:Tracker1_OverVolt_err=0;
    Counter=0;
  state errTrue
    en:Tracker1_OverVolt_err=1;
    Counter=0;
  (default) -> errClear
  errClear -> errConfirm : [TLF35584Tracker1_OverVolt==1]
  errConfirm -> errClear [order 2] : [TLF35584Tracker1_OverVolt==0]
  errTrue -> errClear : [Recover==1]
  errConfirm -> errTrue [order 1] : [Counter >= ti35584err_C]
  data: TLF35584Tracker1_OverVolt input boolean; Tracker1_OverVolt_err output boolean; ti35584err_C input uint16; Counter local uint16; Recover input uint8

== stateflow chart EHB_MOTOR/EHB_MOTOR_PRO/DIAG/TLF35584Diag/ErrorSignalCount5 ==
  state errConfirm
    en:Tracker1_UnderVolt_err=0;
    du:Counter++;
  state errClear
    en:Tracker1_UnderVolt_err=0;
    Counter=0;
  state errTrue
    en:Tracker1_UnderVolt_err=1;
    Counter=0;
  (default) -> errClear
  errClear -> errConfirm : [TLF35584Tracker1_UnderVolt==1]
  errConfirm -> errClear [order 2] : [TLF35584Tracker1_UnderVolt==0]
  errTrue -> errClear : [Recover==1]
  errConfirm -> errTrue [order 1] : [Counter >= ti35584err_C]
  data: TLF35584Tracker1_UnderVolt input boolean; Tracker1_UnderVolt_err output boolean; ti35584err_C input uint16; Counter local uint16; Recover input uint8

== stateflow chart EHB_MOTOR/EHB_MOTOR_PRO/DIAG/TLF35584Diag/ErrorSignalCount6 ==
  state errConfirm
    en:VltRef_Short2GND_err=0;
    du:Counter++;
  state errClear
    en:VltRef_Short2GND_err=0;
    Counter=0;
  state errTrue
    en:VltRef_Short2GND_err=1;
    Counter=0;
  (default) -> errClear
  errClear -> errConfirm : [TLF35584VltRef_Short2GND==1]
  errConfirm -> errClear [order 2] : [TLF35584VltRef_Short2GND==0]
  errTrue -> errClear : [Recover==1]
  errConfirm -> errTrue [order 1] : [Counter >= ti35584err_C]
  data: TLF35584VltRef_Short2GND input boolean; VltRef_Short2GND_err output boolean; ti35584err_C input uint16; Counter local uint16; Recover input uint8

== stateflow chart EHB_MOTOR/EHB_MOTOR_PRO/DIAG/TLF35584Diag/ErrorSignalCount7 ==
  state errConfirm
    en:VltRef_OverVolt_err=0;
    du:Counter++;
  state errClear
    en:VltRef_OverVolt_err=0;
    Counter=0;
  state errTrue
    en:VltRef_OverVolt_err=1;
    Counter=0;
  (default) -> errClear
  errClear -> errConfirm : [TLF35584VltRef_OverVolt==1]
  errConfirm -> errClear [order 2] : [TLF35584VltRef_OverVolt==0]
  errTrue -> errClear : [Recover==1]
  errConfirm -> errTrue [order 1] : [Counter >= ti35584err_C]
  data: TLF35584VltRef_OverVolt input boolean; VltRef_OverVolt_err output boolean; ti35584err_C input uint16; Counter local uint16; Recover input uint8

== stateflow chart EHB_MOTOR/EHB_MOTOR_PRO/DIAG/TLF35584Diag/ErrorSignalCount8 ==
  state errConfirm
    en:VltRef_UnderVolt_err=0;
    du:Counter++;
  state errClear
    en:VltRef_UnderVolt_err=0;
    Counter=0;
  state errTrue
    en:VltRef_UnderVolt_err=1;
    Counter=0;
  (default) -> errClear
  errClear -> errConfirm : [TLF35584VltRef_UnderVolt==1]
  errConfirm -> errClear [order 2] : [TLF35584VltRef_UnderVolt==0]
  errTrue -> errClear : [Recover==1]
  errConfirm -> errTrue [order 1] : [Counter >= ti35584err_C]
  data: TLF35584VltRef_UnderVolt input boolean; VltRef_UnderVolt_err output boolean; ti35584err_C input uint16; Counter local uint16; Recover input uint8

== stateflow chart EHB_MOTOR/EHB_MOTOR_PRO/DIAG/TLF35584Diag/ErrorSignalCount10 ==
  state errConfirm
    en:CommuLDO_OverVolt_err=0;
    du:Counter++;
  state errClear
    en:CommuLDO_OverVolt_err=0;
    Counter=0;
  state errTrue
    en:CommuLDO_OverVolt_err=1;
    Counter=0;
  (default) -> errClear
  errClear -> errConfirm : [TLF35584CommuLDO_OverVolt==1]
  errConfirm -> errClear [order 2] : [TLF35584CommuLDO_OverVolt==0]
  errTrue -> errClear : [Recover==1]
  errConfirm -> errTrue [order 1] : [Counter >= ti35584err_C]
  data: TLF35584CommuLDO_OverVolt input boolean; CommuLDO_OverVolt_err output boolean; ti35584err_C input uint16; Counter local uint16; Recover input uint8

== stateflow chart EHB_MOTOR/EHB_MOTOR_PRO/DIAG/TLF35584Diag/ErrorSignalCount11 ==
  state errConfirm
    en:CommuLDO_UnderVolt_err=0;
    du:Counter++;
  state errClear
    en:CommuLDO_UnderVolt_err=0;
    Counter=0;
  state errTrue
    en:CommuLDO_UnderVolt_err=1;
    Counter=0;
  (default) -> errClear
  errClear -> errConfirm : [TLF35584CommuLDO_UnderVolt==1]
  errConfirm -> errClear [order 2] : [TLF35584CommuLDO_UnderVolt==0]
  errTrue -> errClear : [Recover==1]
  errConfirm -> errTrue [order 1] : [Counter >= ti35584err_C]
  data: TLF35584CommuLDO_UnderVolt input boolean; CommuLDO_UnderVolt_err output boolean; ti35584err_C input uint16; Counter local uint16; Recover input uint8

== stateflow chart EHB_MOTOR/EHB_MOTOR_PRO/DIAG/TLF35584Diag/ErrorSignalCount9 ==
  state errConfirm
    en:CommuLDO_Short2GND_err=0;
    du:Counter++;
  state errClear
    en:CommuLDO_Short2GND_err=0;
    Counter=0;
  state errTrue
    en:CommuLDO_Short2GND_err=1;
    Counter=0;
  (default) -> errClear
  errClear -> errConfirm : [TLF35584CommuLDO_Short2GND==1]
  errConfirm -> errClear [order 2] : [TLF35584CommuLDO_Short2GND==0]
  errTrue -> errClear : [Recover==1]
  errConfirm -> errTrue [order 1] : [Counter >= ti35584err_C]
  data: TLF35584CommuLDO_Short2GND input boolean; CommuLDO_Short2GND_err output boolean; ti35584err_C input uint16; Counter local uint16; Recover input uint8

== stateflow chart EHB_MOTOR/EHB_MOTOR_PRO/DIAG/TLF35584Diag/ErrorSignalCount12 ==
  state errConfirm
    en:CoreVlt_OverVolt_err=0;
    du:Counter++;
  state errClear
    en:CoreVlt_OverVolt_err=0;
    Counter=0;
  state errTrue
    en:CoreVlt_OverVolt_err=1;
    Counter=0;
  (default) -> errClear
  errClear -> errConfirm : [TLF35584CoreVlt_OverVolt==1]
  errConfirm -> errClear [order 2] : [TLF35584CoreVlt_OverVolt==0]
  errTrue -> errClear : [Recover==1]
  errConfirm -> errTrue [order 1] : [Counter >= ti35584err_C]
  data: TLF35584CoreVlt_OverVolt input boolean; CoreVlt_OverVolt_err output boolean; ti35584err_C input uint16; Counter local uint16; Recover input uint8

== stateflow chart EHB_MOTOR/EHB_MOTOR_PRO/DIAG/TLF35584Diag/ErrorSignalCount13 ==
  state errConfirm
    en:CoreVlt_UnderVolt_err=0;
    du:Counter++;
  state errClear
    en:CoreVlt_UnderVolt_err=0;
    Counter=0;
  state errTrue
    en:CoreVlt_UnderVolt_err=1;
    Counter=0;
  (default) -> errClear
  errClear -> errConfirm : [TLF35584CoreVlt_UnderVolt==1]
  errConfirm -> errClear [order 2] : [TLF35584CoreVlt_UnderVolt==0]
  errTrue -> errClear : [Recover==1]
  errConfirm -> errTrue [order 1] : [Counter >= ti35584err_C]
  data: TLF35584CoreVlt_UnderVolt input boolean; CoreVlt_UnderVolt_err output boolean; ti35584err_C input uint16; Counter local uint16; Recover input uint8

== stateflow chart EHB_MOTOR/EHB_MOTOR_PRO/DIAG/TLF35584Diag/ErrorSignalCount14 ==
  state errConfirm
    en:CoreVlt_Short2GND_err=0;
    du:Counter++;
  state errClear
    en:CoreVlt_Short2GND_err=0;
    Counter=0;
  state errTrue
    en:CoreVlt_Short2GND_err=1;
    Counter=0;
  (default) -> errClear
  errClear -> errConfirm : [TLF35584CoreVlt_Short2GND==1]
  errConfirm -> errClear [order 2] : [TLF35584CoreVlt_Short2GND==0]
  errTrue -> errClear : [Recover==1]
  errConfirm -> errTrue [order 1] : [Counter >= ti35584err_C]
  data: TLF35584CoreVlt_Short2GND input boolean; CoreVlt_Short2GND_err output boolean; ti35584err_C input uint16; Counter local uint16; Recover input uint8

== stateflow chart EHB_MOTOR/EHB_MOTOR_PRO/DIAG/TLF35584Diag/ErrorSignalCount15 ==
  state errConfirm
    en:StdbyLDO_OverVolt_err=0;
    du:Counter++;
  state errClear
    en:StdbyLDO_OverVolt_err=0;
    Counter=0;
  state errTrue
    en:StdbyLDO_OverVolt_err=1;
    Counter=0;
  (default) -> errClear
  errClear -> errConfirm : [TLF35584StdbyLDO_OverVolt==1]
  errConfirm -> errClear [order 2] : [TLF35584StdbyLDO_OverVolt==0]
  errTrue -> errClear : [Recover==1]
  errConfirm -> errTrue [order 1] : [Counter >= ti35584err_C]
  data: TLF35584StdbyLDO_OverVolt input boolean; StdbyLDO_OverVolt_err output boolean; ti35584err_C input uint16; Counter local uint16; Recover input uint8

== stateflow chart EHB_MOTOR/EHB_MOTOR_PRO/DIAG/TLF35584Diag/ErrorSignalCount16 ==
  state errConfirm
    en:StdbyLDO_UnderVolt_err=0;
    du:Counter++;
  state errClear
    en:StdbyLDO_UnderVolt_err=0;
    Counter=0;
  state errTrue
    en:StdbyLDO_UnderVolt_err=1;
    Counter=0;
  (default) -> errClear
  errClear -> errConfirm : [TLF35584StdbyLDO_UnderVolt==1]
  errConfirm -> errClear [order 2] : [TLF35584StdbyLDO_UnderVolt==0]
  errTrue -> errClear : [Recover==1]
  errConfirm -> errTrue [order 1] : [Counter >= ti35584err_C]
  data: TLF35584StdbyLDO_UnderVolt input boolean; StdbyLDO_UnderVolt_err output boolean; ti35584err_C input uint16; Counter local uint16; Recover input uint8

== stateflow chart EHB_MOTOR/EHB_MOTOR_PRO/DIAG/TLF35584Diag/ErrorSignalCount17 ==
  state errConfirm
    en:StdbyLDO_Short2GND_err=0;
    du:Counter++;
  state errClear
    en:StdbyLDO_Short2GND_err=0;
    Counter=0;
  state errTrue
    en:StdbyLDO_Short2GND_err=1;
    Counter=0;
  (default) -> errClear
  errClear -> errConfirm : [TLF35584StdbyLDO_Short2GND==1]
  errConfirm -> errClear [order 2] : [TLF35584StdbyLDO_Short2GND==0]
  errTrue -> errClear : [Recover==1]
  errConfirm -> errTrue [order 1] : [Counter >= ti35584err_C]
  data: TLF35584StdbyLDO_Short2GND input boolean; StdbyLDO_Short2GND_err output boolean; ti35584err_C input uint16; Counter local uint16; Recover input uint8

== stateflow chart EHB_MOTOR/EHB_MOTOR_PRO/DIAG/TLF35584Diag/ErrorSignalCount18 ==
  state errConfirm
    en:uCLDO_OverVolt_err=0;
    du:Counter++;
  state errClear
    en:uCLDO_OverVolt_err=0;
    Counter=0;
  state errTrue
    en:uCLDO_OverVolt_err=1;
    Counter=0;
  (default) -> errClear
  errClear -> errConfirm : [TLF35584uCLDO_OverVolt==1]
  errConfirm -> errClear [order 2] : [TLF35584uCLDO_OverVolt==0]
  errTrue -> errClear : [Recover==1]
  errConfirm -> errTrue [order 1] : [Counter >= ti35584err_C]
  data: TLF35584uCLDO_OverVolt input boolean; uCLDO_OverVolt_err output boolean; ti35584err_C input uint16; Counter local uint16; Recover input uint8

== stateflow chart EHB_MOTOR/EHB_MOTOR_PRO/DIAG/TLF35584Diag/ErrorSignalCount19 ==
  state errConfirm
    en:uCLDO_UnderVolt_err=0;
    du:Counter++;
  state errClear
    en:uCLDO_UnderVolt_err=0;
    Counter=0;
  state errTrue
    en:uCLDO_UnderVolt_err=1;
    Counter=0;
  (default) -> errClear
  errClear -> errConfirm : [TLF35584uCLDO_UnderVolt==1]
  errConfirm -> errClear [order 2] : [TLF35584uCLDO_UnderVolt==0]
  errTrue -> errClear : [Recover==1]
  errConfirm -> errTrue [order 1] : [Counter >= ti35584err_C]
  data: TLF35584uCLDO_UnderVolt input boolean; uCLDO_UnderVolt_err output boolean; ti35584err_C input uint16; Counter local uint16; Recover input uint8

== stateflow chart EHB_MOTOR/EHB_MOTOR_PRO/DIAG/TLF35584Diag/ErrorSignalCount20 ==
  state errConfirm
    en:uCLDO_Short2GND_err=0;
    du:Counter++;
  state errClear
    en:uCLDO_Short2GND_err=0;
    Counter=0;
  state errTrue
    en:uCLDO_Short2GND_err=1;
    Counter=0;
  (default) -> errClear
  errClear -> errConfirm : [TLF35584uCLDO_Short2GND==1]
  errConfirm -> errClear [order 2] : [TLF35584uCLDO_Short2GND==0]
  errTrue -> errClear : [Recover==1]
  errConfirm -> errTrue [order 1] : [Counter >= ti35584err_C]
  data: TLF35584uCLDO_Short2GND input boolean; uCLDO_Short2GND_err output boolean; ti35584err_C input uint16; Counter local uint16; Recover input uint8

== stateflow chart EHB_MOTOR/EHB_MOTOR_PRO/DIAG/TLF35584Diag/ErrorSignalCount21 ==
  state errConfirm
    en:PreVolt_OverVolt_err=0;
    du:Counter++;
  state errClear
    en:PreVolt_OverVolt_err=0;
    Counter=0;
  state errTrue
    en:PreVolt_OverVolt_err=1;
    Counter=0;
  (default) -> errClear
  errClear -> errConfirm : [TLF35584PreVolt_OverVolt==1]
  errConfirm -> errClear [order 2] : [TLF35584PreVolt_OverVolt==0]
  errTrue -> errClear : [Recover==1]
  errConfirm -> errTrue [order 1] : [Counter >= ti35584err_C]
  data: TLF35584PreVolt_OverVolt input boolean; PreVolt_OverVolt_err output boolean; ti35584err_C input uint16; Counter local uint16; Recover input uint8

== stateflow chart EHB_MOTOR/EHB_MOTOR_PRO/DIAG/TLF35584Diag/ErrorSignalCount22 ==
  state errConfirm
    en:PreVolt_UnderVolt_err=0;
    du:Counter++;
  state errClear
    en:PreVolt_UnderVolt_err=0;
    Counter=0;
  state errTrue
    en:PreVolt_UnderVolt_err=1;
    Counter=0;
  (default) -> errClear
  errClear -> errConfirm : [TLF35584PreVolt_UnderVolt==1]
  errConfirm -> errClear [order 2] : [TLF35584PreVolt_UnderVolt==0]
  errTrue -> errClear : [Recover==1]
  errConfirm -> errTrue [order 1] : [Counter >= ti35584err_C]
  data: TLF35584PreVolt_UnderVolt input boolean; PreVolt_UnderVolt_err output boolean; ti35584err_C input uint16; Counter local uint16; Recover input uint8

== stateflow chart EHB_MOTOR/EHB_MOTOR_PRO/DIAG/TLF35584Diag/ErrorSignalCount23 ==
  state errConfirm
    en:PreVolt_Short2GND_err=0;
    du:Counter++;
  state errClear
    en:PreVolt_Short2GND_err=0;
    Counter=0;
  state errTrue
    en:PreVolt_Short2GND_err=1;
    Counter=0;
  (default) -> errClear
  errClear -> errConfirm : [TLF35584PreVolt_Short2GND==1]
  errConfirm -> errClear [order 2] : [TLF35584PreVolt_Short2GND==0]
  errTrue -> errClear : [Recover==1]
  errConfirm -> errTrue [order 1] : [Counter >= ti35584err_C]
  data: TLF35584PreVolt_Short2GND input boolean; PreVolt_Short2GND_err output boolean; ti35584err_C input uint16; Counter local uint16; Recover input uint8

== stateflow chart EHB_MOTOR/EHB_MOTOR_PRO/INPUT/DI/Debounce ==
  state none
    en:cnt_0=0;
    cnt_1=0;
    none -> (junction 63)
    (junction 63) -> (junction 49) [order 1] : [input>0]
    (junction 63) -> (junction 58) [order 2]
    (junction 49) -> (junction 60)
    (junction 58) -> (junction 62) [order 1] : [cnt_0>=50]
    (junction 60) -> (junction 54) [order 1] : [cnt_1>=50]
    (junction 62) -> (junction 47) : {output=0;
        | cnt_0=0;
        | cnt_1=0;}
    (junction 58) -> (junction 68) [order 2] : {cnt_0=cnt_0+1;
        | cnt_1=0;}
    (junction 60) -> (junction 66) [order 2] : {cnt_1=cnt_1+1;
        | cnt_0=0;}
    (junction 54) -> (junction 56) : {output=1;
        | cnt_0=0;
        | cnt_1=0;}
    (junction 47) -> (junction 68)
    (junction 66) -> (junction 68)
    (junction 56) -> (junction 66)
  (default) -> none
  data: cnt_0 local uint8 size=1; output output boolean size=1; input input; cnt_1 local uint8 size=1

== stateflow chart EHB_MOTOR/EHB_MOTOR_PRO/INPUT/DI/Debounce1 ==
  state none
    en:cnt_0=0;
    cnt_1=0;
    none -> (junction 63)
    (junction 63) -> (junction 49) [order 1] : [input>0]
    (junction 63) -> (junction 58) [order 2]
    (junction 49) -> (junction 60)
    (junction 58) -> (junction 62) [order 1] : [cnt_0>=2]
    (junction 60) -> (junction 54) [order 1] : [cnt_1>=2]
    (junction 62) -> (junction 47) : {output=0;
        | cnt_0=0;
        | cnt_1=0;}
    (junction 58) -> (junction 68) [order 2] : {cnt_0=cnt_0+1;}
    (junction 60) -> (junction 66) [order 2] : {cnt_1=cnt_1+1;}
    (junction 54) -> (junction 56) : {output=1;
        | cnt_0=0;
        | cnt_1=0;}
    (junction 47) -> (junction 68)
    (junction 66) -> (junction 68)
    (junction 56) -> (junction 66)
  (default) -> none
  data: cnt_0 local uint8 size=1; output output boolean size=1; input input; cnt_1 local uint8 size=1

== stateflow chart EHB_MOTOR/EHB_MOTOR_PRO/INPUT/DI/Debounce2 ==
  state none
    en:cnt_0=0;
    cnt_1=0;
    none -> (junction 63)
    (junction 63) -> (junction 49) [order 1] : [input>0]
    (junction 63) -> (junction 58) [order 2]
    (junction 49) -> (junction 60)
    (junction 58) -> (junction 62) [order 1] : [cnt_0>=2]
    (junction 60) -> (junction 54) [order 1] : [cnt_1>=2]
    (junction 62) -> (junction 47) : {output=0;
        | cnt_0=0;
        | cnt_1=0;}
    (junction 58) -> (junction 68) [order 2] : {cnt_0=cnt_0+1;}
    (junction 60) -> (junction 66) [order 2] : {cnt_1=cnt_1+1;}
    (junction 54) -> (junction 56) : {output=1;
        | cnt_0=0;
        | cnt_1=0;}
    (junction 47) -> (junction 68)
    (junction 66) -> (junction 68)
    (junction 56) -> (junction 66)
  (default) -> none
  data: cnt_0 local uint8 size=1; output output boolean size=1; input input; cnt_1 local uint8 size=1

== stateflow chart EHB_MOTOR/EHB_MOTOR_PRO/INPUT/DI/Debounce3 ==
  state none
    en:cnt_0=0;
    cnt_1=0;
    none -> (junction 63)
    (junction 63) -> (junction 49) [order 1] : [input>0]
    (junction 63) -> (junction 58) [order 2]
    (junction 49) -> (junction 60)
    (junction 58) -> (junction 62) [order 1] : [cnt_0>=2]
    (junction 60) -> (junction 54) [order 1] : [cnt_1>=2]
    (junction 62) -> (junction 47) : {output=0;
        | cnt_0=0;
        | cnt_1=0;}
    (junction 58) -> (junction 68) [order 2] : {cnt_0=cnt_0+1;}
    (junction 60) -> (junction 66) [order 2] : {cnt_1=cnt_1+1;}
    (junction 54) -> (junction 56) : {output=1;
        | cnt_0=0;
        | cnt_1=0;}
    (junction 47) -> (junction 68)
    (junction 66) -> (junction 68)
    (junction 56) -> (junction 66)
  (default) -> none
  data: cnt_0 local uint8 size=1; output output boolean size=1; input input; cnt_1 local uint8 size=1

== stateflow chart EHB_MOTOR/EHB_MOTOR_PRO/INPUT/DI/Debounce4 ==
  state none
    en:cnt_0=0;
    cnt_1=0;
    none -> (junction 63)
    (junction 63) -> (junction 49) [order 1] : [input>0]
    (junction 63) -> (junction 58) [order 2]
    (junction 49) -> (junction 60)
    (junction 58) -> (junction 62) [order 1] : [cnt_0>=2]
    (junction 60) -> (junction 54) [order 1] : [cnt_1>=2]
    (junction 62) -> (junction 47) : {output=0;
        | cnt_0=0;
        | cnt_1=0;}
    (junction 58) -> (junction 68) [order 2] : {cnt_0=cnt_0+1;}
    (junction 60) -> (junction 66) [order 2] : {cnt_1=cnt_1+1;}
    (junction 54) -> (junction 56) : {output=1;
        | cnt_0=0;
        | cnt_1=0;}
    (junction 47) -> (junction 68)
    (junction 66) -> (junction 68)
    (junction 56) -> (junction 66)
  (default) -> none
  data: cnt_0 local uint8 size=1; output output boolean size=1; input input; cnt_1 local uint8 size=1

== stateflow chart EHB_MOTOR/EHB_MOTOR_PRO/INPUT/DI/Debounce5 ==
  state none
    en:cnt_0=0;
    cnt_1=0;
    none -> (junction 63)
    (junction 63) -> (junction 49) [order 1] : [input>0]
    (junction 63) -> (junction 58) [order 2]
    (junction 49) -> (junction 60)
    (junction 58) -> (junction 62) [order 1] : [cnt_0>=2]
    (junction 60) -> (junction 54) [order 1] : [cnt_1>=2]
    (junction 62) -> (junction 47) : {output=0;
        | cnt_0=0;
        | cnt_1=0;}
    (junction 58) -> (junction 68) [order 2] : {cnt_0=cnt_0+1;}
    (junction 60) -> (junction 66) [order 2] : {cnt_1=cnt_1+1;}
    (junction 54) -> (junction 56) : {output=1;
        | cnt_0=0;
        | cnt_1=0;}
    (junction 47) -> (junction 68)
    (junction 66) -> (junction 68)
    (junction 56) -> (junction 66)
  (default) -> none
  data: cnt_0 local uint8 size=1; output output boolean size=1; input input; cnt_1 local uint8 size=1

== stateflow chart EHB_MOTOR/EHB_MOTOR_PRO/INPUT/DI/Debounce6 ==
  state none
    en:cnt_0=0;
    cnt_1=0;
    none -> (junction 63)
    (junction 63) -> (junction 49) [order 1] : [input>0]
    (junction 63) -> (junction 58) [order 2]
    (junction 49) -> (junction 60)
    (junction 58) -> (junction 62) [order 1] : [cnt_0>=2]
    (junction 60) -> (junction 54) [order 1] : [cnt_1>=2]
    (junction 62) -> (junction 47) : {output=0;
        | cnt_0=0;
        | cnt_1=0;}
    (junction 58) -> (junction 68) [order 2] : {cnt_0=cnt_0+1;}
    (junction 60) -> (junction 66) [order 2] : {cnt_1=cnt_1+1;}
    (junction 54) -> (junction 56) : {output=1;
        | cnt_0=0;
        | cnt_1=0;}
    (junction 47) -> (junction 68)
    (junction 66) -> (junction 68)
    (junction 56) -> (junction 66)
  (default) -> none
  data: cnt_0 local uint8 size=1; output output boolean size=1; input input; cnt_1 local uint8 size=1
